simulink model "b_controller_secure"  (R2018b)
settings: Solver=ode45  StartTime=0.0  StopTime=10  RelTol=1e-3  EnableMultiTasking=on
undefined symbols (not defined in the file): Tab, Tba, Tca, Tcb
settings Model: Creator=Luan Nguyen  LastModifiedBy=gautam
settings DataIOCC: LimitDataPoints=on  SaveFormat=Array  SignalLoggingSaveFormat=ModelDataLogs
settings OptimizationCC: ExpressionDepthLimit=2147483647  LifeSpan=inf
settings DebuggingCC: UnderspecifiedInitializationDetection=Classic  MergeDetectMultiDrivingBlocksExec=none  IgnoredZcDiagnostic=none  MultiTaskDSMMsg=warning  MultiTaskCondExecSysMsg=none  StateNameClashWarn=warning  SFUnexpectedBacktrackingDiag=warning  SFNoUnconditionalDefaultTransitionDiag=warning  SFExecutionAtInitializationDiag=none
settings HardwareCC: ProdBitPerPointer=32  ProdBitPerSizeT=32  ProdBitPerPtrDiffT=32  ProdLargestAtomicFloat=None  ProdIntDivRoundTo=Undefined  ProdEndianess=Unspecified  ProdWordSize=32  ProdHWDeviceType=32-bit Generic
settings ModelReferenceCC: PropagateSignalLabelsOutOfModel=off
settings SFSimCC: SimUseLocalCustomCode=off
settings RTWCC: RTWUseLocalCustomCode=off
settings CodeAppCC: StateflowObjectComments=on
settings GRTTargetCC: TargetLangStandard=C89/C90 (ANSI)  GeneratePreprocessorConditionals=Disable all
settings ConfigComp: CovMetricSettings=dw  CovHtmlReporting=on  CovSaveCumulativeToWorkspaceVar=on  CovSaveSingleToWorkspaceVar=on  CovExternalEMLEnable=off  CovSFcnEnable=off

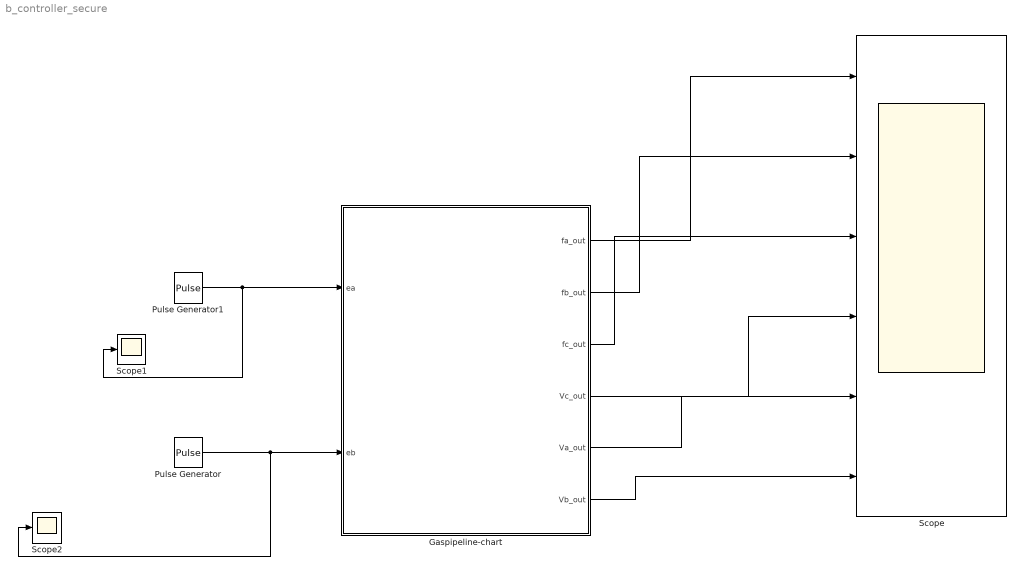
== system b_controller_secure ==
  Gaspipeline-chart : Stateflow chart  TreatAsAtomicUnit=on
  Pulse Generator : DiscretePulseGenerator  PulseType=Time based  Amplitude=3  Period=10
  Pulse Generator1 : DiscretePulseGenerator  PulseType=Time based  Amplitude=-3  Period=10
  Scope : Scope  NumInputPorts=6
  Scope1 : Scope
  Scope2 : Scope
  wires:
  Gaspipeline-chart/1(fa_out) -> Scope/1
  Gaspipeline-chart/2(fb_out) -> Scope/2
  Gaspipeline-chart/3(fc_out) -> Scope/3
  Gaspipeline-chart/4(Vc_out) -> Scope/4
  Gaspipeline-chart/5(Va_out) -> Scope/5
  Gaspipeline-chart/6(Vb_out) -> Scope/6
  Pulse Generator1/1 -> Scope1/1, Gaspipeline-chart/1(ea)
  Pulse Generator/1 -> Scope2/1, Gaspipeline-chart/2(eb)

== stateflow chart b_controller_secure/Gaspipeline-chart ==
  settings: updateMethod=CONTINUOUS
  state ModeB1
    du:
    Va_dot = fa; Va_out = Va; fa_dot = 0; fa_out = fa;
    Vb_dot = fb; Vb_out = Vb; fb_dot = 0; fb_out = fb;
    Vc_dot = fc; Vc_out = Vc; fc_dot = 0; fc_out = fc;
  state ModeB3
    du:
    zb_dot = 1;
    Va_dot = fa; Va_out = Va; fa_dot = 0; fa_out = fa;
    Vb_dot = fb; Vb_out = Vb; fb_dot = 0; fb_out = fb;
    Vc_dot = fc; Vc_out = Vc; fc_dot = 0; fc_out = fc;
  state ModeB5
    du:
    zb_dot = 1;
    Va_dot = fa; Va_out = Va; fa_dot = 0; fa_out = ea;
    Vb_dot = fb; Vb_out = Vb; fb_dot = 0; fb_out = fb;
    Vc_dot = fc; Vc_out = Vc; fc_dot = 0; fc_out = fc;
  ModeB3 -> ModeB1 : [zb >= Tba]
      | {fb = fb+tmpB; zb = 0;}
  (default) -> ModeB1 : {fb = 5; fc = 10; fa = 5; zb = 0; tmpB = 0;}
  ModeB1 -> ModeB3 [order 1] : [eb >= 0]{tmpB = eb;zb = 0;}
  ModeB1 -> ModeB5 [order 2] : [eb <= 0 ]
      | {tmpB = eb;zb = 0;}
  ModeB5 -> ModeB1 : [zb >= 1]
      | {fb = fb+ tmpB;zb = 0;}
  data: za local double; zb local double; fa local double; fa_out output double; ea input double; fb local double; fb_out output double; fc local double; fc_out output double; Va local double; Vb local double; Vc local double; Vc_out output double; Va_out output double; Vb_out output double; Tba parameter double; Tca parameter double; Tcb parameter double; eb input double; Tab parameter double; zc local double; tmpA local double; tmpB local double; tmpC local double
  data za settings: updateMethod=SF_CONTINUOUS_TIME_DATA
  data zb settings: updateMethod=SF_CONTINUOUS_TIME_DATA
  data fa settings: updateMethod=SF_CONTINUOUS_TIME_DATA
  data fb settings: updateMethod=SF_CONTINUOUS_TIME_DATA
  data fc settings: updateMethod=SF_CONTINUOUS_TIME_DATA
  data Va settings: updateMethod=SF_CONTINUOUS_TIME_DATA
  data Vb settings: updateMethod=SF_CONTINUOUS_TIME_DATA
  data Vc settings: updateMethod=SF_CONTINUOUS_TIME_DATA
  data zc settings: updateMethod=SF_CONTINUOUS_TIME_DATA
